simulink model "modeloferpid"  (R2022b)
settings: Solver=ode4  StartTime=0.0  StopTime=360  FixedStep=0.25  RelTol=1e-3
libraries: slpidlib x1
settings Model: Creator=DELL  LastModifiedBy=DELL

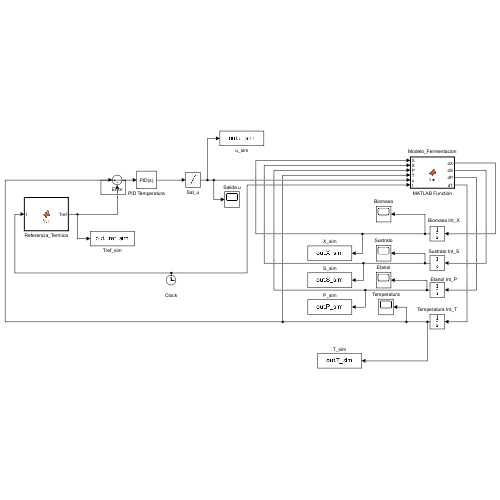
[thumbnail: Simulink's stored preview of the top-level diagram]
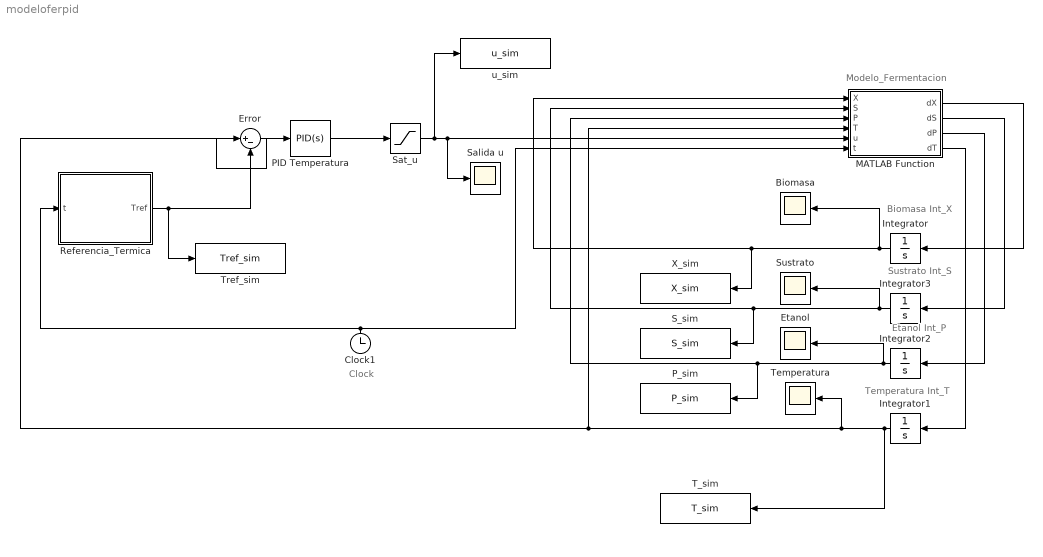
== system modeloferpid ==
  note: Modelo_Fermentacion
  note: Clock
  note: Temperatura Int_T
  note: Etanol Int_P
  note: Sustrato Int_S
  note: Biomasa Int_X
  Biomasa : Scope
  Clock1 : Clock
  Error : Sum  Inputs=|+-
  Etanol : Scope
  Integrator : Integrator  InitialCondition=1
  Integrator1 : Integrator  InitialCondition=10
  Integrator2 : Integrator
  Integrator3 : Integrator  InitialCondition=140
  MATLAB Function : MATLAB Function  Tag=Modelo_Fermentacion  TreatAsAtomicUnit=on
  PID Temperatura : slpidlib/PID Controller  Controller=PID  Form=Parallel  TimeDomain=Continuous-time  UseExternalTs=off  SampleTime=-1  IntegratorMethod=Forward Euler  FilterMethod=Forward Euler  ControllerParametersSource=internal  P=0.90  I=0.08  UseKiTs=off  D=0.02  N=100  UseFilter=on  TunerSelectOption=Transfer Function Based (PID Tuner App)  InitialConditionSource=internal  InitialConditionForIntegrator=0  InitialConditionForFilter=0  DifferentiatorICPrevScaledInput=0  ExternalReset=none  TrackingMode=off  Kt=1  LimitOutput=off  SatLimitsSource=internal  UpperSaturationLimit=inf  LowerSaturationLimit=-inf  LinearizeAsGain=on  AntiWindupMode=none  Kb=1  LimitIntegrator=off  UpperIntegratorSaturationLimit=inf  LowerIntegratorSaturationLimit=-inf  POutMin=[]  POutMax=[]  IOutMin=[]  IOutMax=[]  DOutMin=[]  DOutMax=[]  NOutMin=[]  NOutMax=[]  SumOutMin=[]  SumOutMax=[]  SaturationOutMin=[]  SaturationOutMax=[]  PParamMin=[]  PParamMax=[]  IParamMin=[]  IParamMax=[]  DParamMin=[]  DParamMax=[]  NParamMin=[]  NParamMax=[]  KbParamMin=[]  KbParamMax=[]  KtParamMin=[]  KtParamMax=[]  KbOutMin=[]  KbOutMax=[]  KtOutMin=[]  KtOutMax=[]  IntegratorOutMin=[]  IntegratorOutMax=[]  FilterOutMin=[]  FilterOutMax=[]  SumI1OutMin=[]  SumI1OutMax=[]  SumI2OutMin=[]  SumI2OutMax=[]  SumI3OutMin=[]  SumI3OutMax=[]  SumI4OutMin=[]  SumI4OutMax=[]  SumDOutMin=[]  SumDOutMax=[]  DifferentiatorOutMin=[]  DifferentiatorOutMax=[]  FilterDiffOutCoefMin=[]  FilterDiffOutCoefMax=[]  ReciprocalOutMin=[]  ReciprocalOutMax=[]  SumDenOutMin=[]  SumDenOutMax=[]  SumNumOutMin=[]  SumNumOutMax=[]  DivideOutMin=[]  DivideOutMax=[]  UdiffTsProdOutMin=[]  UdiffTsProdOutMax=[]  NTsProdOutMin=[]  NTsProdOutMax=[]  UintegralTsProdOutMin=[]  UintegralTsProdOutMax=[]  UngainTsProdOutMin=[]  UngainTsProdOutMax=[]  ClampingZeroOutDataTypeStr=Inherit: Inherit via back propagation  ClampingZeroOutMin=[]  ClampingZeroOutMax=[]  FilterDenConstantOutDataTypeStr=Inherit: Inherit via back propagation  FilterDenConstantOutMin=[]  FilterDenConstantOutMax=[]  PCopyOutDataTypeStr=Inherit: Inherit via back propagation  PCopyOutMin=[]  PCopyOutMax=[]  NCopyOutDataTypeStr=Inherit: Inherit via back propagation  NCopyOutMin=[]  NCopyOutMax=[]  IntegratorContinuousStateAttributes=''  IntegratorStateMustResolveToSignalObject=off  IntegratorRTWStateStorageClass=Auto  FilterContinuousStateAttributes=''  FilterStateMustResolveToSignalObject=off  FilterRTWStateStorageClass=Auto  ParallelPVariant=InternalParameters  IdealPVariant=Disabled  IVariant=InternalParameters  DVariant=InternalParameters  IntegratorVariant=Continuous  SatVariant=Disabled  AWVariant=Passthrough  PCopyVariant=Disabled  TRVariant=Disabled  FdbkBlocksVariant=Forward  IdealPFdbkVariant=Disabled  SatFdbkVariant=Disabled  DerivativeFilterVariant=ContFilter  NVariant=InternalParameters  NCopyVariant=Disabled  FilterICVariant=InternalICsFilter  IntegratorICVariant=InternalICs  ExternalResetVariant=Disabled  TRSumVariant=Passthrough  SumFdbkVariant=Disabled  SumVariant=Sum_PID  TsampFilterVariant=InternalTs  TsampNgainVariant=Passthrough  TsampIntegralVariant=Passthrough  ExternalSaturationOutDataTypeStr=Inherit: Same as second input
  P_sim : ToWorkspace  VariableName=P_sim  SaveFormat=Structure With Time  SampleTime=-1
  Referencia_Termica : MATLAB Function  Tag=Modelo_Fermentacion  TreatAsAtomicUnit=on
  S_sim : ToWorkspace  VariableName=S_sim  SaveFormat=Structure With Time  SampleTime=-1
  Salida u : Scope
      settings: Tag=Temperatura
  Sat_u : Saturate  Tag=Sat_u  UpperLimit=1  LowerLimit=0
  Sustrato : Scope
  T_sim : ToWorkspace  VariableName=T_sim  SaveFormat=Structure With Time  SampleTime=-1
  Temperatura : Scope
      settings: Tag=Temperatura
  Tref_sim : ToWorkspace  VariableName=Tref_sim  SaveFormat=Structure With Time  SampleTime=-1
  X_sim : ToWorkspace  VariableName=X_sim  SaveFormat=Structure With Time  SampleTime=-1
  u_sim : ToWorkspace  VariableName=u_sim  SaveFormat=Structure With Time  SampleTime=-1
  wires:
  Error/1 -> PID Temperatura/1
  PID Temperatura/1 -> Sat_u/1
  MATLAB Function/1(dX) -> Integrator/1
  MATLAB Function/2(dS) -> Integrator3/1
  MATLAB Function/3(dP) -> Integrator2/1
  MATLAB Function/4(dT) -> Integrator1/1
  Sat_u/1 -> u_sim/1, Salida u/1, MATLAB Function/5(u)
  Integrator/1 -> Biomasa/1, X_sim/1, MATLAB Function/1(X)
  Integrator3/1 -> Sustrato/1, S_sim/1, MATLAB Function/2(S)
  Integrator2/1 -> Etanol/1, P_sim/1, MATLAB Function/3(P)
  Integrator1/1 -> T_sim/1, Temperatura/1, Error/1, MATLAB Function/4(T)
  Referencia_Termica/1(Tref) -> Tref_sim/1, Error/2
  Clock1/1 -> MATLAB Function/6(t), Referencia_Termica/1(t)

== matlab function modeloferpid/Referencia_Termica ==
  data: Tref output; t input
function Tref = fcn(t)
% Referencia térmica para fermentación + maduración tipo pilsen/lager
% Proceso total: 15 días = 360 h
% Fermentación: 5 días = 120 h
% Maduración: 10 días = 240 h

if t <= 24
    % Día 0 a 1: subida de 10 a 12 °C
    Tref = 10 + (12 - 10)*(t/24);

elseif t <= 72
    % Día 1 a 3: mantener 12 °C
    Tref = 12;

elseif t <= 96
    % Día 3 a 4: subida de 12 a 14 °C
    Tref = 12 + (14 - 12)*((t - 72)/24);

elseif t <= 120
    % Día 4 a 5: mantener 14 °C
    Tref = 14;

elseif t <= 144
    % Día 5 a 6: enfriamiento de 14 a -1.5 °C
    Tref = 14 + (-1.5 - 14)*((t - 120)/24);

else
    % Día 6 a 15: maduración fría a -1.5 °C
    Tref = -1.5;
end

== matlab function modeloferpid/MATLAB Function ==
  data: X input; S input; P input; T input; u input; dX output; t input; dS output; dP output; dT output
function [dX,dS,dP,dT] = fcn(X,S,P,T,u,t)

% Modelo dinámico simplificado para fermentación + maduración cervecera
% Perfil tipo pilsen/lager en TCC

%% Parámetros cinéticos ajustados

mu_max = 0.030;     % 1/h, tasa máxima ajustada
Ks     = 10;        % g/L
Yxs    = 0.25;      % gX/gS
Yps    = 0.45;      % gP/gS

%% Parámetros térmicos

alpha  = 0.08;      % generación térmica por consumo de sustrato
beta   = 1.20;      % capacidad máxima de enfriamiento [°C/h]
Tamb   = 20;        % temperatura ambiente [°C]
k_env  = 0.02;      % intercambio térmico con ambiente [1/h]

%% Extracto residual

Sres = 28;          % g/L, extracto residual aproximado

%% Protección numérica

if X < 0
    X = 0;
end

if S < Sres
    S = Sres;
end

%% Sustrato fermentable disponible

Sf = max(S - Sres, 0);

%% Factor térmico de actividad fermentativa

if T < 2
    fT = 0.05;
elseif T < 6
    fT = 0.30;
else
    fT = 1.00;
end

%% Cinética tipo Monod modificada

mu = fT * mu_max * Sf/(Ks + Sf + eps);

%% Balances de masa

dX = mu*X;

dS = -(1/Yxs)*mu*X;

% Evitar que el sustrato baje del residual
if S <= Sres && dS < 0
    dS = 0;
end

dP = Yps*(-dS);

%% Balance térmico

Qgen  = alpha*(-dS);       % calor generado por fermentación
Qcool = beta*u;            % enfriamiento
Qenv  = k_env*(Tamb - T);  % intercambio térmico con ambiente

%% Perturbación térmica en Simulink

% Por ahora sin perturbación dentro del bloque.
% Si deseas luego agregamos perturbaciones por tramo.
d = 0;

dT = Qgen - Qcool + Qenv + d;
